simulink model "PreCharge"  (R2022b)
settings: Solver=FixedStepDiscrete  StartTime=0.0  StopTime=10.0  FixedStep=0.0001  RelTol=1e-3
undefined symbols (not defined in the file or in its folder): ParamCfg_ChargeEnable_u16, ParamCfg_PrechargeUdc_u16
settings Model: DataDictionary=MCU_PreCharge.sldd  Creator=ZYH  LastModifiedBy=ZYH
settings OptimizationCC: DefaultParameterBehavior=Inlined  EnhancedBackFolding=on  PassReuseOutputArgsAs=Individual arguments  ZeroExternalMemoryAtStartup=off  ZeroInternalMemoryAtStartup=off  OptimizeBlockOrder=speed  DifferentSizesBufferReuse=on  OptimizationCustomize=off  EfficientTunableParamExpr=on
settings DebuggingCC: ParameterTunabilityLossMsg=error
settings SFSimCC: MATLABDynamicMemAlloc=off
settings RTWCC: Description=Embedded Coder  SystemTargetFile=ert.tlc  GenCodeOnly=on  TemplateMakefile=ert_default_tmf
settings CodeAppCC: ForceParamTrailComments=on  IgnoreCustomStorageClasses=off  OperatorAnnotations=on  SimulinkDataObjDesc=on  SFDataObjDesc=on  InsertBlockDesc=on
settings ERTTargetCC: TargetLangStandard=C99 (ISO)  GenerateSampleERTMain=on  InlinedParameterPlacement=NonHierarchical  ERTCustomFileTemplate=example_file_process.tlc

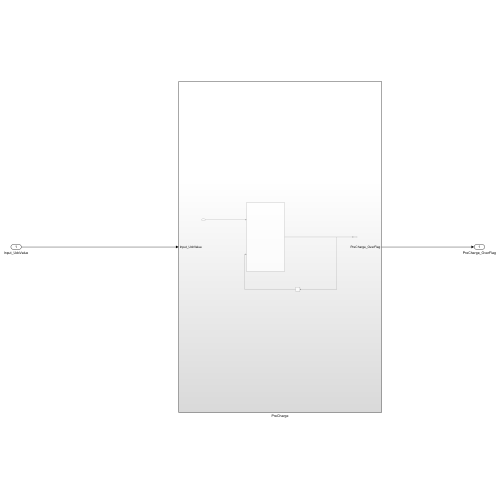
[thumbnail: Simulink's stored preview of the top-level diagram]
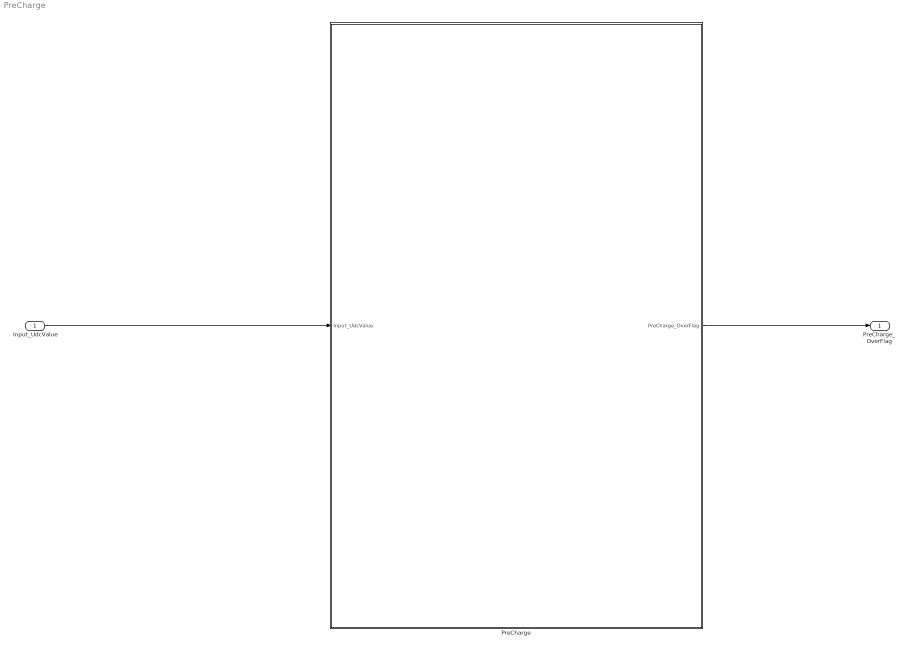
== system PreCharge ==
  Input_UdcValue : Inport
  PreCharge : Subsystem
  PreCharge_OverFlag : Outport
  wires:
  Input_UdcValue/1 -> PreCharge/1(Input_UdcValue)
  PreCharge/1(PreCharge_OverFlag) -> PreCharge_OverFlag/1

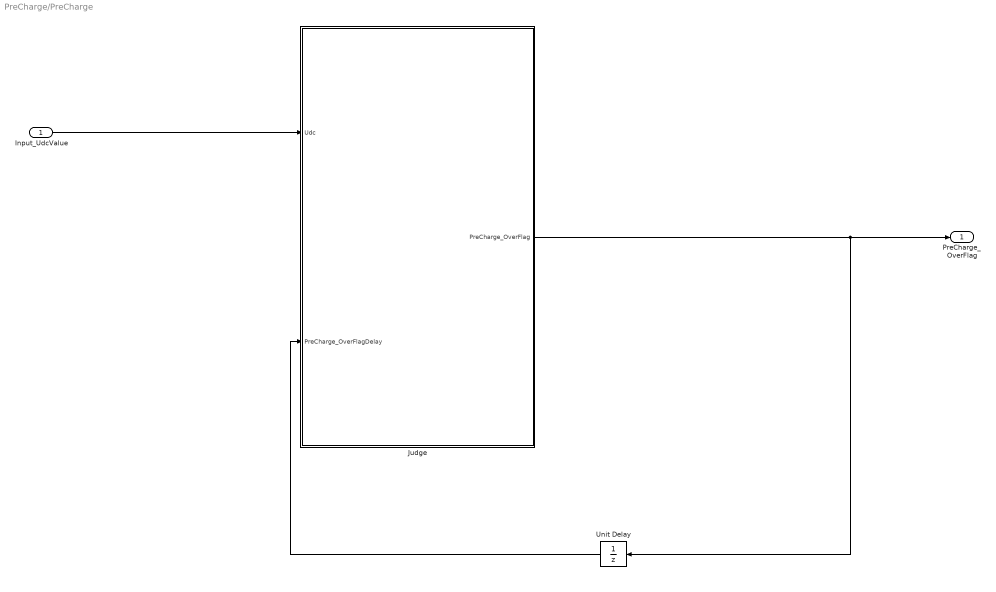
== system PreCharge/PreCharge ==
  Input_UdcValue : Inport
  Judge : Subsystem
  Unit Delay : UnitDelay  SampleTime=-1  HasFrameUpgradeWarning=on
  PreCharge_OverFlag : Outport
  wires:
  Judge/1(PreCharge_OverFlag) -> Unit Delay/1, PreCharge_OverFlag/1
  Unit Delay/1 -> Judge/2(PreCharge_OverFlagDelay)
  Input_UdcValue/1 -> Judge/1(Udc)

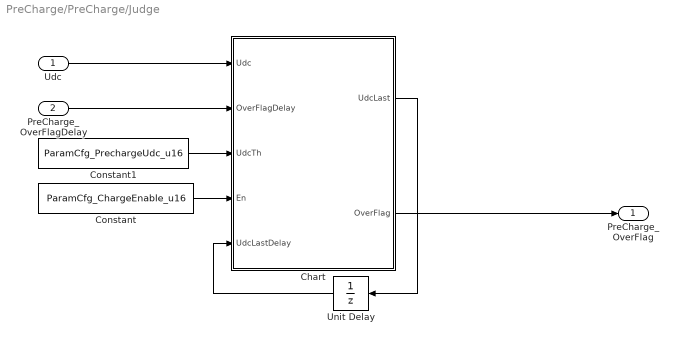
== system PreCharge/PreCharge/Judge ==
  Udc : Inport
  PreCharge_OverFlagDelay : Inport  Port=2
  Chart : Stateflow chart  TreatAsAtomicUnit=on
  Constant : Constant  Value=ParamCfg_ChargeEnable_u16
  Constant1 : Constant  Value=ParamCfg_PrechargeUdc_u16
  Unit Delay : UnitDelay  SampleTime=-1  HasFrameUpgradeWarning=on
  PreCharge_OverFlag : Outport
  wires:
  PreCharge_OverFlagDelay/1 -> Chart/2(OverFlagDelay)
  Udc/1 -> Chart/1(Udc)
  Constant1/1 -> Chart/3(UdcTh)
  Constant/1 -> Chart/4(En)
  Chart/1(UdcLast) -> Unit Delay/1
  Unit Delay/1 -> Chart/5(UdcLastDelay)
  Chart/2(OverFlag) -> PreCharge_OverFlag/1

== stateflow chart PreCharge/Judge/Chart ==
  (default) -> (junction 4)
  (junction 4) -> (junction 7) : [En == true && OverFlagDelay ==0]
  (junction 7) -> (junction 9) : [Udc > UdcTh]
  (junction 9) -> (junction 11) [order 1] : [Udc-UdcLast<5]
  (junction 11) -> (junction 13) [order 1] : {PreCntTime = PreCntTime + 1}
  (junction 9) -> (junction 27) [order 2]
  (junction 11) -> (junction 22) [order 2] : {
      | PreCntTime = 0;
      | UdcLast = Udc
      | }
  (junction 13) -> (junction 17) : [PreCntTime >=100]
  (junction 17) -> (junction 19) : {
      | PreCntTime = 0;
      | OverFlag = 1
      | }
  (junction 19) -> (junction 24)
  (junction 22) -> (junction 27)
  (junction 24) -> (junction 22)
  (junction 27) -> (junction 30)
  data: Udc input; OverFlagDelay input; UdcTh input; En input; UdcLast output double; PreCntTime local uint16 =0; OverFlag output uint8 =0; UdcLastDelay input
